simulink model "TORA"  (R2019b)
settings: Solver=VariableStepAuto  StartTime=0.0  StopTime=50.0  RelTol=1e-3
settings Model: Creator=Administrator  LastModifiedBy=Administrator

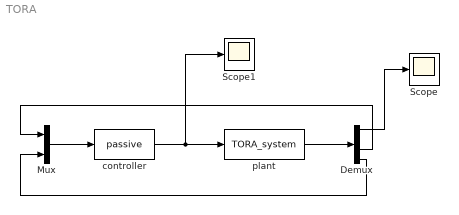
== system TORA ==
  Demux : Demux
  Mux : Mux  Inputs=2
  Scope : Scope
  Scope1 : Scope
  controller : S-Function  FunctionName=passive  SFunctionDeploymentMode=off  EnableBusSupport=off
  plant : S-Function  FunctionName=TORA_system  SFunctionDeploymentMode=off  EnableBusSupport=off
  wires:
  controller/1 -> Scope1/1, plant/1
  plant/1 -> Demux/1
  Demux/1 -> Scope/1
  Mux/1 -> controller/1
  Demux/3 -> Mux/1
  Demux/4 -> Mux/2
